simulink model "SF028A_AssiHiFrq"  (R2013b)
settings: Solver=FixedStepDiscrete  SolverMode=SingleTasking  StartTime=0.0  StopTime=1  FixedStep=0.002  RelTol=1e-3
undefined symbols (not defined in the file): ARCHGLBPRM_2MILLISEC_SEC_F32
libraries: FixdToFloat x4, FloatToFixd x4, Fil x3, BilnrIntrpnMplX x3, NxtrAbslt x1, NxtrMath x1, NxtrLim x1, LnrIntrpn x1, simulink x1
Description:
  | This function provides a means of compensating for system inertia and road feedback.  It is
  |  tunable over both vehicle speed and handwheel torque to obtain the desired level of disurbance
  |  rejection under various operating conditions.  It passes handwheel torque through a high-pass
  |  filter and multiplies the resulting signal by a tunable gain factor.  The output is known as
  |  high-frequency assist and is simply added to the usual assist calculated elsewhere.
settings Model: Creator=lzz0tm  LastModifiedBy=XZB1DB
settings Model: ModifiedHistory=|
  | 001
  | Initial release
  | K. Derry
  | 3-Nov-2011
  | n/a
  | 
  | 002
  | Use common vehicle speed table from SF-00
  | Reduce Torq tables from 32x16 to 13x12
  | Eliminate filter cutoff frequency WIR blending
  | Update to floating point high pass filter.
  | Changed filter cutoff required resolution from 0.005 Hz to 0.125 Hz.
  | Renamed 2-D cal tables from '...t..' to '..t2..' format.
  | Redefined display variables.
  | Eliminate Word doc.
  | K. Derry
  | 13-Mar-2013
  | ICR-4006
settings SolverCC: AutoInsertRateTranBlk=on  InsertRTBMode=Always
settings DataIOCC: LimitDataPoints=off  SaveFormat=Structure  ReturnWorkspaceOutputs=on
settings OptimizationCC: BlockReduction=off  InlineParams=on  ZeroExternalMemoryAtStartup=off  ZeroInternalMemoryAtStartup=off  OptimizeModelRefInitCode=on  LifeSpan=1
settings DebuggingCC: ConsistencyChecking=warning  ArrayBoundsChecking=warning  SignalInfNanChecking=error  SignalRangeChecking=warning  UnderspecifiedInitializationDetection=Simplified  SolverPrmCheckMsg=error  InheritedTsInSrcMsg=error  DiscreteInheritContinuousMsg=error  SingleTaskRateTransMsg=error  TasksWithSamePriorityMsg=error  SigSpecEnsureSampleTimeMsg=error  CheckMatrixSingularityMsg=error  ParameterUnderflowMsg=error  ParameterPrecisionLossMsg=error  ParameterTunabilityLossMsg=error  FixptConstUnderflowMsg=warning  FixptConstOverflowMsg=warning  VectorMatrixConversionMsg=error  SignalLabelMismatchMsg=error  UnconnectedInputMsg=error  UnconnectedOutputMsg=error  UnconnectedLineMsg=error  SFcnCompatibilityMsg=error  UniqueDataStoreMsg=warning  BusObjectLabelMismatch=error  RootOutportRequireBusObject=error  AssertControl=DisableAll  ModelReferenceIOMsg=error  ModelReferenceVersionMismatchMessage=warning  ModelReferenceIOMismatchMessage=error  ModelReferenceCSMismatchMessage=warning  ModelReferenceDataLoggingMessage=error  StateNameClashWarn=warning  StrictBusMsg=ErrorOnBusTreatedAsVector  NonBusSignalsTreatedAsBus=error  SFUnexpectedBacktrackingDiag=error  SFInvalidInputDataAccessInChartInitDiag=error  SFNoUnconditionalDefaultTransitionDiag=error  SFTransitionOutsideNaturalParentDiag=error  SFUnconditionalTransitionShadowingDiag=error  SFUndirectedBroadcastEventsDiag=error
settings ModelReferenceCC: ModelReferenceNumInstancesAllowed=Single
settings RTWCC: SystemTargetFile=autosar.tlc  GenCodeOnly=on  TemplateMakefile=ert_default_tmf  Description=AUTOSAR  GenerateReport=on  ProcessScript=autosar_make_rtw_hook  LaunchReport=on
settings CodeAppCC: GenerateComments=off  IgnoreCustomStorageClasses=off  CustomSymbolStrType=$N$R$M  CustomSymbolStrBlkIO=$N$M  SimulinkBlockComments=off
settings STFCustomTargetCC: ParMdlRefBuildCompliant=on  CompOptLevelCompliant=on  IncludeMdlTerminateFcn=off  CombineOutputUpdateFcns=on  SuppressErrorStatus=on  ERTFirstTimeCompliant=on  ERTCustomFileBanners=on  SupportNonFinite=off  SupportComplex=off  SupportContinuousTime=off  SupportNonInlinedSFcns=off  MATLABClassNameForMDSCustomization=Simulink.SoftwareTarget.ERTCustomization  AutosarCompliant=on  GRTInterface=off  SystemTargetFile=autosar.tlc
settings ERTTargetCC: CodeReplacementLibrary=ANSI_C  ConcurrentExecutionCompliant=off  IncludeMdlTerminateFcn=off  SuppressErrorStatus=on  SupportNonFinite=off  SupportComplex=off  ModelStepFunctionPrototypeControlCompliant=off  CPPClassGenCompliant=off  AutosarCompliant=on  InlinedParameterPlacement=NonHierarchical  ERTCustomFileTemplate=example_file_process.tlc  EnableUserReplacementTypes=on

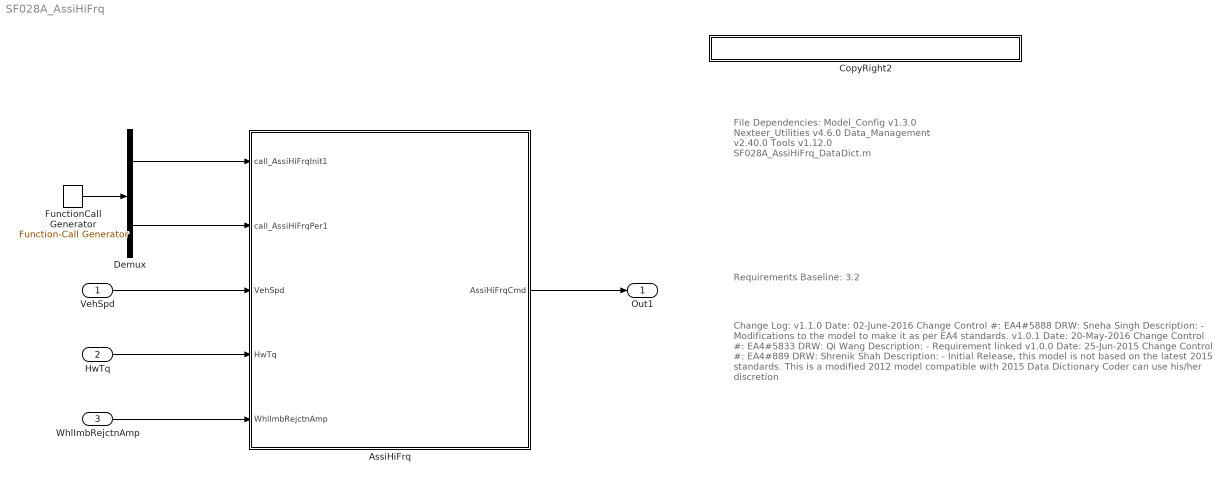
== system SF028A_AssiHiFrq ==
  note: File Dependencies:
      |
      | Model_Config v1.3.0
      | Nexteer_Utilities v4.6.0
      | Data_Management v2.40.0
      | Tools v1.12.0
      | SF028A_AssiHiFrq_DataDict.m
  note: Requirements Baseline: 3.2
  note: Change Log:
      |
      | v1.1.0
      | Date: 02-June-2016
      | Change Control #: EA4#5888
      | DRW: Sneha Singh
      | Description:
      | - Modifications to the model to make it as per EA4 standards.
      |
      | v1.0.1
      | Date: 20-May-2016
      | Change Control #: EA4#5833
      | DRW:  Qi Wang
      | Description:
      | - Requirement linked
      |
      | v1.0.0
      | Date: 25-Jun-2015
      | Change Control #: EA4#889
      | DRW:  Shrenik Shah
      | Description:
      | - Initial Release, this model is not based on the latest 2015 standards.
      |   This is a modified 2012 model compatible with 2015 Data Dictionary
      |   Coder can use his/her discretion
  VehSpd : Inport  RequirementInfo={} %GIDa_a0d763e6_ccd7_4f6b_982f_233123faece6
  HwTq : Inport  RequirementInfo={} %GIDa_23d74bf2_0b4b_4fb1_b85a_9dd0076d3e89  Port=2
  WhlImbRejctnAmp : Inport  RequirementInfo={} %GIDa_98bbb477_aef9_404c_9caf_7c83616077f3  Port=3
  AssiHiFrq : Subsystem
  CopyRight2 : Subsystem  Description=|  mask(Copyright Information){none=on}
      | Copyright info block.                                               
      |                                                                     
      | Place copyright information at the top of every subsystem in design.
      mask prompts: none "No parameters"
      mask help: Place copyright information at the top of every subsystem in design.
      mask Display:
      | NxtrConf = 'Nexteer Confidential';
      | 
      | sys = bdroot; %handle for the current model ("system")
      | first = get_param(sys,'Created');
      | if(isempty(first))
      |     first = datestr(now,'yyyy');
      | else
      |     first = first(end-3:end);  %year is last four digits
      | end
      | 
      | last = get_param(sys,'LastModifiedDate');
      | if isempty(last)
      |     last = datestr(now,'yyyy');
      | else
      |     last = last(end-3:end);
      | end
      | 
      | if strcmp(first,last)
      |     fprintf('%s -- Copyright %s Nexteer',NxtrConf,first)
      | else
      |     fprintf('%s -- %s%s- %s Nexteer',NxtrConf,char(169),first,last)
      | end
  Demux : Demux  Outputs=2
  FunctionCall Generator : simulink/Ports & Subsystems/Function-Call Generator  sample_time=0.002  numberOfIterations=1
  Out1 : Outport
  wires:
  VehSpd/1 -> AssiHiFrq/3(VehSpd)
  AssiHiFrq/1(AssiHiFrqCmd) -> Out1/1
  Demux/2 -> AssiHiFrq/2(call_AssiHiFrqPer1)
  Demux/1 -> AssiHiFrq/1(call_AssiHiFrqInit1)
  HwTq/1 -> AssiHiFrq/4(HwTq)
  WhlImbRejctnAmp/1 -> AssiHiFrq/5(WhlImbRejctnAmp)
  FunctionCall Generator/1 -> Demux/1

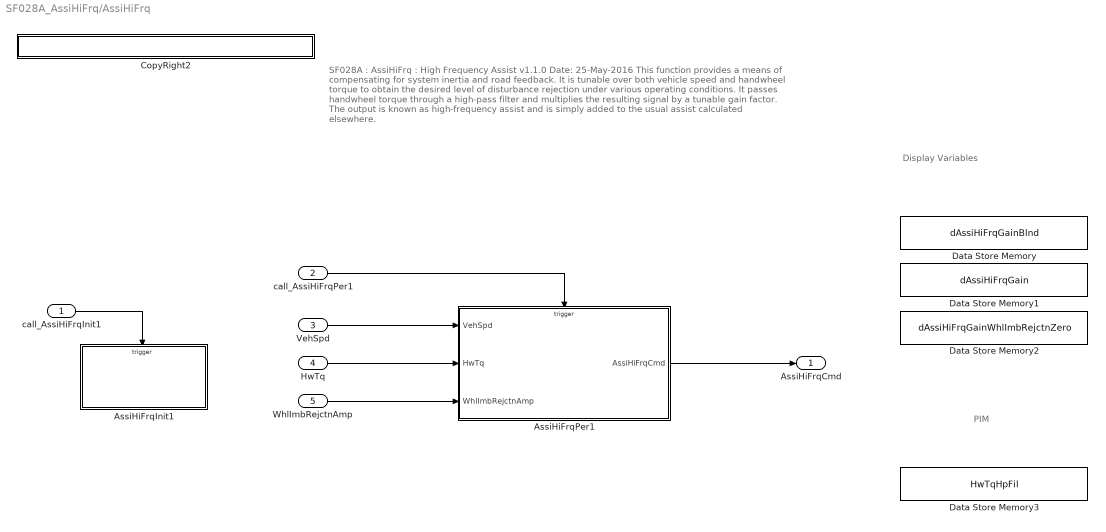
== system SF028A_AssiHiFrq/AssiHiFrq ==
  note: SF028A : AssiHiFrq : High Frequency Assist
      | v1.1.0
      | Date: 25-May-2016
      |
      |   This function provides a means of compensating for system inertia and
      |   road feedback. It is tunable over both vehicle speed and handwheel torque
      |   to obtain the desired level of disturbance rejection under various operating
      |   conditions. It passes handwheel torque through a high-pass filter and multiplies
      |   the resulting signal by a tunable gain factor. The output is known as high-frequency
      |   assist and is simply added to the usual assist calculated elsewhere.
  note: Display Variables
  note: PIM
  call_AssiHiFrqInit1 : Inport
  call_AssiHiFrqPer1 : Inport  Port=2
  VehSpd : Inport  RequirementInfo={'linktype_rmi_doors' '0000a536 (/E-STEER Core/SubSystem Specifications/Application Functions/SF028A High Frequency Assist)' '#SF028A_9' 'true' 'REQ:SF028A_9' '' } %GIDa_86218aeb_648a_47e3_8b98_4acdbc8753c3  Port=3
  HwTq : Inport  RequirementInfo={'linktype_rmi_doors' '0000a536 (/E-STEER Core/SubSystem Specifications/Application Functions/SF028A High Frequency Assist)' '#SF028A_32' 'true' 'REQ:SF028A_32' '' } %GIDa_018f3a3f_b6e0_4310_ba85_9c867fd20861  Port=4
  WhlImbRejctnAmp : Inport  RequirementInfo={'linktype_rmi_doors' '0000a536 (/E-STEER Core/SubSystem Specifications/Application Functions/SF028A High Frequency Assist)' '#SF028A_33' 'true' 'REQ:SF028A_33' '' } %GIDa_1ed4b7fa_c4c1_41ae_86ab_75f4c7c6c1a1  Port=5
  AssiHiFrqInit1 : Subsystem
  AssiHiFrqPer1 : Subsystem
  CopyRight2 : Subsystem  Description=|  mask(Copyright Information){none=on}
      | Copyright info block.                                               
      |                                                                     
      | Place copyright information at the top of every subsystem in design.
      mask prompts: none "No parameters"
      mask help: Place copyright information at the top of every subsystem in design.
      mask Display:
      | NxtrConf = 'Nexteer Confidential';
      | 
      | sys = bdroot; %handle for the current model ("system")
      | first = get_param(sys,'Created');
      | if(isempty(first))
      |     first = datestr(now,'yyyy');
      | else
      |     first = first(end-3:end);  %year is last four digits
      | end
      | 
      | last = get_param(sys,'LastModifiedDate');
      | if isempty(last)
      |     last = datestr(now,'yyyy');
      | else
      |     last = last(end-3:end);
      | end
      | 
      | if strcmp(first,last)
      |     fprintf('%s -- Copyright %s Nexteer',NxtrConf,first)
      | else
      |     fprintf('%s -- %s%s- %s Nexteer',NxtrConf,char(169),first,last)
      | end
  Data Store Memory : DataStoreMemory  DataStoreName=dAssiHiFrqGainBlnd  ReadBeforeWriteMsg=warning  WriteAfterWriteMsg=warning  WriteAfterReadMsg=warning  StateMustResolveToSignalObject=on
  Data Store Memory1 : DataStoreMemory  DataStoreName=dAssiHiFrqGain  ReadBeforeWriteMsg=warning  WriteAfterWriteMsg=warning  WriteAfterReadMsg=warning  StateMustResolveToSignalObject=on
  Data Store Memory2 : DataStoreMemory  DataStoreName=dAssiHiFrqGainWhlImbRejctnZero  ReadBeforeWriteMsg=warning  WriteAfterWriteMsg=warning  WriteAfterReadMsg=warning  StateMustResolveToSignalObject=on
  Data Store Memory3 : DataStoreMemory  DataStoreName=HwTqHpFil  ReadBeforeWriteMsg=warning  WriteAfterWriteMsg=warning  WriteAfterReadMsg=warning  InitialValue=[]  OutDataTypeStr=Bus: FilHpRec1  StateMustResolveToSignalObject=on
  AssiHiFrqCmd : Outport  RequirementInfo={'linktype_rmi_doors' '0000a536 (/E-STEER Core/SubSystem Specifications/Application Functions/SF028A High Frequency Assist)' '#SF028A_11' 'true' 'REQ:SF028A_11' '' } %GIDa_e9edc8ae_1989_4889_b077_85200aef58b1
  wires:
  VehSpd/1 -> AssiHiFrqPer1/1(VehSpd)
  HwTq/1 -> AssiHiFrqPer1/2(HwTq)
  WhlImbRejctnAmp/1 -> AssiHiFrqPer1/3(WhlImbRejctnAmp)
  AssiHiFrqPer1/1(AssiHiFrqCmd) -> AssiHiFrqCmd/1
  call_AssiHiFrqInit1/1 -> AssiHiFrqInit1/Trigger
  call_AssiHiFrqPer1/1 -> AssiHiFrqPer1/Trigger

== system SF028A_AssiHiFrq/CopyRight2 ==

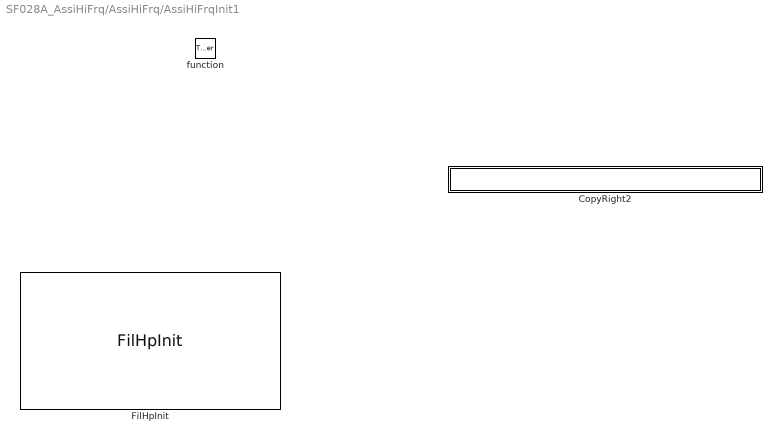
== system SF028A_AssiHiFrq/AssiHiFrq/AssiHiFrqInit1 ==
  function : TriggerPort  TriggerType=function-call
  CopyRight2 : Subsystem  Description=|  mask(Copyright Information){none=on}
      | Copyright info block.                                               
      |                                                                     
      | Place copyright information at the top of every subsystem in design.
      mask prompts: none "No parameters"
      mask help: Place copyright information at the top of every subsystem in design.
      mask Display:
      | NxtrConf = 'Nexteer Confidential';
      | 
      | sys = bdroot; %handle for the current model ("system")
      | first = get_param(sys,'Created');
      | if(isempty(first))
      |     first = datestr(now,'yyyy');
      | else
      |     first = first(end-3:end);  %year is last four digits
      | end
      | 
      | last = get_param(sys,'LastModifiedDate');
      | if isempty(last)
      |     last = datestr(now,'yyyy');
      | else
      |     last = last(end-3:end);
      | end
      | 
      | if strcmp(first,last)
      |     fprintf('%s -- Copyright %s Nexteer',NxtrConf,first)
      | else
      |     fprintf('%s -- %s%s- %s Nexteer',NxtrConf,char(169),first,last)
      | end
  FilHpInit : Fil/FilHpInit  Ic=0  Ts=ARCHGLBPRM_2MILLISEC_SEC_F32  Freq=AssiHiFrqHpFilFrq  StVar=HwTqHpFil

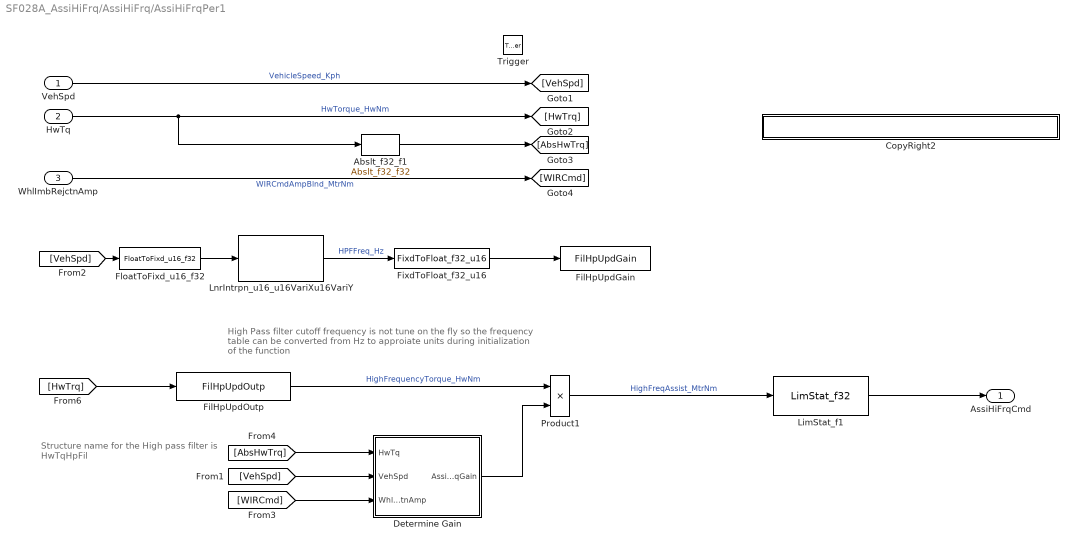
== system SF028A_AssiHiFrq/AssiHiFrq/AssiHiFrqPer1 ==
  note: Structure name for the High pass filter is
      | HwTqHpFil
  note: High Pass filter cutoff frequency is not tune on the fly
      | so the frequency table can be converted from Hz to approiate units
      | during initialization of the function
  VehSpd : Inport
  HwTq : Inport  Port=2
  WhlImbRejctnAmp : Inport  Port=3
  Trigger : TriggerPort  TriggerType=function-call
  Abslt_f32_f1 : NxtrAbslt/Abslt_f32_f32  SFunctionSpec=single y1 = Abslt_f32_f32(single u1)
      settings: AttributesFormatString=%<Name>
  CopyRight2 : Subsystem  Description=|  mask(Copyright Information){none=on}
      | Copyright info block.                                               
      |                                                                     
      | Place copyright information at the top of every subsystem in design.
      mask prompts: none "No parameters"
      mask help: Place copyright information at the top of every subsystem in design.
      mask Display:
      | NxtrConf = 'Nexteer Confidential';
      | 
      | sys = bdroot; %handle for the current model ("system")
      | first = get_param(sys,'Created');
      | if(isempty(first))
      |     first = datestr(now,'yyyy');
      | else
      |     first = first(end-3:end);  %year is last four digits
      | end
      | 
      | last = get_param(sys,'LastModifiedDate');
      | if isempty(last)
      |     last = datestr(now,'yyyy');
      | else
      |     last = last(end-3:end);
      | end
      | 
      | if strcmp(first,last)
      |     fprintf('%s -- Copyright %s Nexteer',NxtrConf,first)
      | else
      |     fprintf('%s -- %s%s- %s Nexteer',NxtrConf,char(169),first,last)
      | end
  Determine Gain : Subsystem  RequirementInfo={'linktype_rmi_doors' '0000a536 (/E-STEER Core/SubSystem Specifications/Application Functions/SF028A High Frequency Assist)' '#SF028A_43' 'true' 'REQ:SF028A_43' '' } %GIDa_af960609_91e3_43c5_ab4d_107c7baa9860
  FilHpUpdGain : Fil/FilHpUpdGain  RequirementInfo={'linktype_rmi_doors' '0000a536 (/E-STEER Core/SubSystem Specifications/Application Functions/SF028A High Frequency Assist)' '#SF028A_41' 'true' 'REQ:SF028A_41' '' } %GIDa_8e3b42aa_8642_4651_9b6a_418eb8f56bc0  Priority=1  Ts=ARCHGLBPRM_2MILLISEC_SEC_F32  StVar=HwTqHpFil
      link override Data Store Write: DataStoreName=HwTqHpFil  DataStoreElements=HwTqHpFil.CorrnFac
      link override FilLpUpdGain/Data Store Write: DataStoreName=HwTqHpFil  DataStoreElements=HwTqHpFil.FilLpRec.FilGain
      settings: AttributesFormatString=|
      | Ts: %<Ts>
      | StVar: %<StVar>
      | Priority: %<Priority>
  FilHpUpdOutp : Fil/FilHpUpdOutp  RequirementInfo={'linktype_rmi_doors' '0000a536 (/E-STEER Core/SubSystem Specifications/Application Functions/SF028A High Frequency Assist)' '#SF028A_41' 'true' 'REQ:SF028A_41' '' } %GIDa_1df2c897_81de_4861_ba6f_77641fcb59d9  Priority=2  StVar=HwTqHpFil
      link override FilLpUpdOutp/Data Store Write: DataStoreName=HwTqHpFil  DataStoreElements=HwTqHpFil.FilLpRec.FilSt
      settings: AttributesFormatString=|
      | StVar: %<StVar>
      | Priority: %<Priority>
  FixdToFloat_f32_u16 : FixdToFloat/FixdToFloat_f32_u16  RequirementInfo={'linktype_rmi_doors' '0000a536 (/E-STEER Core/SubSystem Specifications/Application Functions/SF028A High Frequency Assist)' '#SF028A_41' 'true' 'REQ:SF028A_41' '' } %GIDa_db33af83_53a0_4c38_8bab_e9aab62ab3c8  Param1=9
  FloatToFixd_u16_f32 : FloatToFixd/FloatToFixd_u16_f32  RequirementInfo={'linktype_rmi_doors' '0000a536 (/E-STEER Core/SubSystem Specifications/Application Functions/SF028A High Frequency Assist)' '#SF028A_41' 'true' 'REQ:SF028A_41' '' } %GIDa_f0a9e907_0e2f_4322_865f_387fb8594bc0  Param1=7
  LimStat_f1 : NxtrLim/LimStat_f32  RequirementInfo={'linktype_rmi_doors' '0000a536 (/E-STEER Core/SubSystem Specifications/Application Functions/SF028A High Frequency Assist)' '#SF028A_63' 'true' 'REQ:SF028A_63' '' } %GIDa_0f16c8b0_219d_4e19_9a4e_83030087b48a  LoLim=SYSGLBPRM_MOTTQCMDLOLIM_MOTNWTMTR_F32  HiLim=SYSGLBPRM_MOTTQCMDHILIM_MOTNWTMTR_F32
      settings: AttributesFormatString=|
      | Low Limit: %<LoLim>
      | High Limit:%<HiLim>
  LnrIntrpn_u16_u16VariXu16VariY : LnrIntrpn/LnrIntrpn_u16_u16VariXu16VariY  RequirementInfo={'linktype_rmi_doors' '0000a536 (/E-STEER Core/SubSystem Specifications/Application Functions/SF028A High Frequency Assist)' '#SF028A_41' 'true' 'REQ:SF028A_41' '' } %GIDa_dffca385_9f8b_4af2_b446_2938b81cfe70  XTbl=SysGlbPrmVehSpdBilnrSeln  YTbl=AssiHiFrqHpFilFrqY
      settings: AttributesFormatString=Lnr ( u16VariX , u16VariY )
  Product1 : Product  RequirementInfo={'linktype_rmi_doors' '0000a536 (/E-STEER Core/SubSystem Specifications/Application Functions/SF028A High Frequency Assist)' '#SF028A_40' 'true' 'REQ:SF028A_40' '' } %GIDa_93c24833_bd88_4de1_a5f6_48da5dfbf139  OutDataTypeStr=single  SaturateOnIntegerOverflow=on  InputSameDT=on
  AssiHiFrqCmd : Outport
  wires:
  Product1/1 -> LimStat_f1/1  "HighFreqAssist_MtrNm"
  VehSpd/1 -> [VehSpd]  "VehicleSpeed_Kph"
  HwTq/1 -> Abslt_f32_f1/1, [HwTrq]  "HwTorque_HwNm"
  WhlImbRejctnAmp/1 -> [WIRCmd]  "WIRCmdAmpBlnd_MtrNm"
  FilHpUpdOutp/1 -> Product1/1  "HighFrequencyTorque_HwNm"
  Determine Gain/1(AssiHiFrqGain) -> Product1/2
  [VehSpd] -> FloatToFixd_u16_f32/1
  [AbsHwTrq] -> Determine Gain/1(HwTq)
  [VehSpd] -> Determine Gain/2(VehSpd)
  [WIRCmd] -> Determine Gain/3(WhlImbRejctnAmp)
  [HwTrq] -> FilHpUpdOutp/1
  LnrIntrpn_u16_u16VariXu16VariY/1 -> FixdToFloat_f32_u16/1  "HPFFreq_Hz"
  LimStat_f1/1 -> AssiHiFrqCmd/1
  FloatToFixd_u16_f32/1 -> LnrIntrpn_u16_u16VariXu16VariY/1
  FixdToFloat_f32_u16/1 -> FilHpUpdGain/1
  Abslt_f32_f1/1 -> [AbsHwTrq]

== system SF028A_AssiHiFrq/AssiHiFrq/CopyRight2 ==

== system SF028A_AssiHiFrq/AssiHiFrq/AssiHiFrqInit1/CopyRight2 ==

== system SF028A_AssiHiFrq/AssiHiFrq/AssiHiFrqPer1/CopyRight2 ==

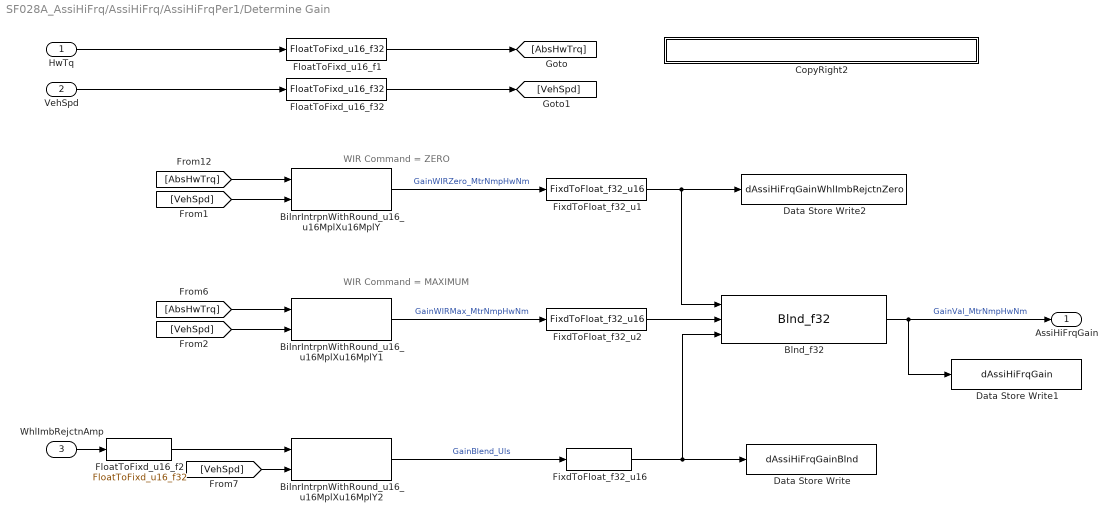
== system SF028A_AssiHiFrq/AssiHiFrq/AssiHiFrqPer1/Determine Gain ==
  note: WIR Command = ZERO
  note: WIR Command = MAXIMUM
  HwTq : Inport
  VehSpd : Inport  Port=2
  WhlImbRejctnAmp : Inport  Port=3
  BilnrIntrpnWithRound_u16_u16MplXu16MplY : BilnrIntrpnMplX/BilnrIntrpnWithRound_u16_u16MplXu16MplY  MplXTbl=AssiHiFrqTqX  MplYTbl=AssiHiFrqGainY  BilnrSelnTbl=SysGlbPrmVehSpdBilnrSeln
      settings: AttributesFormatString=|
      | Bilnr ( u16MplX , u16MplY )
      | XTbl: %<MplXTbl>
      | YTbl: %<MplYTbl>
      | BilnrSelnTbl: %<BilnrSelnTbl>
  BilnrIntrpnWithRound_u16_u16MplXu16MplY1 : BilnrIntrpnMplX/BilnrIntrpnWithRound_u16_u16MplXu16MplY  MplXTbl=AssiHiFrqTqWhlImbRejctnTqX  MplYTbl=AssiHiFrqWhlImbRejctnGainY  BilnrSelnTbl=SysGlbPrmVehSpdBilnrSeln
      settings: AttributesFormatString=|
      | Bilnr ( u16MplX , u16MplY )
      | XTbl: %<MplXTbl>
      | YTbl: %<MplYTbl>
      | BilnrSelnTbl: %<BilnrSelnTbl>
  BilnrIntrpnWithRound_u16_u16MplXu16MplY2 : BilnrIntrpnMplX/BilnrIntrpnWithRound_u16_u16MplXu16MplY  MplXTbl=AssiHiFrqWhlImbRejctnBlndX  MplYTbl=AssiHiFrqWhlImbRejctnBlndY  BilnrSelnTbl=SysGlbPrmVehSpdBilnrSeln
      settings: AttributesFormatString=|
      | Bilnr ( u16MplX , u16MplY )
      | XTbl: %<MplXTbl>
      | YTbl: %<MplYTbl>
      | BilnrSelnTbl: %<BilnrSelnTbl>
  Blnd_f32 : NxtrMath/Blnd_f32  SFunctionSpec=single y1 = Blnd_f32(single u1, single u2, single u3)  Parameter3=on
      settings: AttributesFormatString=%<Name>
  CopyRight2 : Subsystem  Description=|  mask(Copyright Information){none=on}
      | Copyright info block.                                               
      |                                                                     
      | Place copyright information at the top of every subsystem in design.
      mask prompts: none "No parameters"
      mask help: Place copyright information at the top of every subsystem in design.
      mask Display:
      | NxtrConf = 'Nexteer Confidential';
      | 
      | sys = bdroot; %handle for the current model ("system")
      | first = get_param(sys,'Created');
      | if(isempty(first))
      |     first = datestr(now,'yyyy');
      | else
      |     first = first(end-3:end);  %year is last four digits
      | end
      | 
      | last = get_param(sys,'LastModifiedDate');
      | if isempty(last)
      |     last = datestr(now,'yyyy');
      | else
      |     last = last(end-3:end);
      | end
      | 
      | if strcmp(first,last)
      |     fprintf('%s -- Copyright %s Nexteer',NxtrConf,first)
      | else
      |     fprintf('%s -- %s%s- %s Nexteer',NxtrConf,char(169),first,last)
      | end
  Data Store Write : DataStoreWrite  DataStoreName=dAssiHiFrqGainBlnd
  Data Store Write1 : DataStoreWrite  DataStoreName=dAssiHiFrqGain
  Data Store Write2 : DataStoreWrite  DataStoreName=dAssiHiFrqGainWhlImbRejctnZero
  FixdToFloat_f32_u1 : FixdToFloat/FixdToFloat_f32_u16  Param1=13
  FixdToFloat_f32_u16 : FixdToFloat/FixdToFloat_f32_u16  Param1=15
  FixdToFloat_f32_u2 : FixdToFloat/FixdToFloat_f32_u16  Param1=13
  FloatToFixd_u16_f1 : FloatToFixd/FloatToFixd_u16_f32  Param1=11
  FloatToFixd_u16_f2 : FloatToFixd/FloatToFixd_u16_f32  Param1=11
  FloatToFixd_u16_f32 : FloatToFixd/FloatToFixd_u16_f32  Param1=7
  AssiHiFrqGain : Outport
  wires:
  [AbsHwTrq] -> BilnrIntrpnWithRound_u16_u16MplXu16MplY/1
  [VehSpd] -> BilnrIntrpnWithRound_u16_u16MplXu16MplY/2
  [AbsHwTrq] -> BilnrIntrpnWithRound_u16_u16MplXu16MplY1/1
  [VehSpd] -> BilnrIntrpnWithRound_u16_u16MplXu16MplY1/2
  BilnrIntrpnWithRound_u16_u16MplXu16MplY2/1 -> FixdToFloat_f32_u16/1  "GainBlend_Uls"
  BilnrIntrpnWithRound_u16_u16MplXu16MplY/1 -> FixdToFloat_f32_u1/1  "GainWIRZero_MtrNmpHwNm"
  Blnd_f32/1 -> AssiHiFrqGain/1, Data Store Write1/1  "GainVal_MtrNmpHwNm"
  BilnrIntrpnWithRound_u16_u16MplXu16MplY1/1 -> FixdToFloat_f32_u2/1  "GainWIRMax_MtrNmpHwNm"
  [VehSpd] -> BilnrIntrpnWithRound_u16_u16MplXu16MplY2/2
  WhlImbRejctnAmp/1 -> FloatToFixd_u16_f2/1
  HwTq/1 -> FloatToFixd_u16_f1/1
  FixdToFloat_f32_u1/1 -> Blnd_f32/1, Data Store Write2/1
  FixdToFloat_f32_u2/1 -> Blnd_f32/2
  FixdToFloat_f32_u16/1 -> Data Store Write/1, Blnd_f32/3
  FloatToFixd_u16_f2/1 -> BilnrIntrpnWithRound_u16_u16MplXu16MplY2/1
  VehSpd/1 -> FloatToFixd_u16_f32/1
  FloatToFixd_u16_f1/1 -> [AbsHwTrq]
  FloatToFixd_u16_f32/1 -> [VehSpd]

== system SF028A_AssiHiFrq/AssiHiFrq/AssiHiFrqPer1/Determine Gain/CopyRight2 ==
